simulink model "BoostConverter11_5V_616976422"  (R2017a)
settings: Solver=VariableStepAuto  StartTime=0.0  StopTime=0.1  MaxStep=1e-4  RelTol=1e-3
undefined symbols (not defined in the file): Imag, Real
libraries: powerlib x12
settings Model: Creator=Weliwaththa's - ROG  LastModifiedBy=Weliwaththa's - ROG

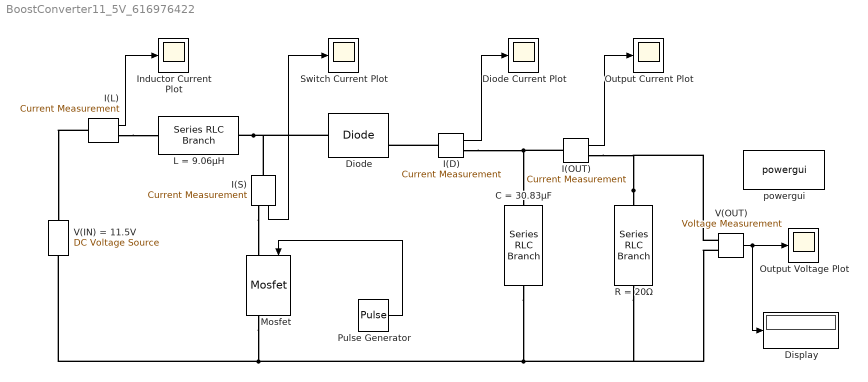
== system BoostConverter11_5V_616976422 ==
  C = 30.83µF : powerlib/Elements/Series RLC Branch  LConnTagsString=__new0  RConnTagsString=__new0  BranchType=C  Resistance=1  Inductance=1e-3  SetiL0=off  InitialCurrent=0  Capacitance=30.83e-6  Setx0=off  InitialVoltage=0  Measurements=None
  Diode : powerlib/Power Electronics/Diode  Ron=0.001  Lon=0  Vf=0.8  IC=0  UseSnubber=0  Rs=500  Cs=250e-9  Measurements=on
  Diode Current Plot : Scope
  Display : Display
  I(D) : powerlib/Measurements/Current Measurement  PhasorSimulation=off  OutputType=Complex  PSBequivalent=0
  I(L) : powerlib/Measurements/Current Measurement  PhasorSimulation=off  OutputType=Real-Imag  PSBequivalent=0
  I(OUT) : powerlib/Measurements/Current Measurement  PhasorSimulation=off  OutputType=Complex  PSBequivalent=0
  I(S) : powerlib/Measurements/Current Measurement  PhasorSimulation=off  OutputType=Complex  PSBequivalent=0
  Inductor Current Plot : Scope
  L = 9.06µH : powerlib/Elements/Series RLC Branch  LConnTagsString=__new0  RConnTagsString=__new0  BranchType=L  Resistance=1  Inductance=9.06e-6  SetiL0=off  InitialCurrent=0  Capacitance=1e-6  Setx0=off  InitialVoltage=0  Measurements=None
  Mosfet : powerlib/Power Electronics/Mosfet  Ron=0  Lon=0  Rd=0  Vfd=0  IC=0  Rs=1e5  Cs=inf  Measurements=on
  Output Current Plot : Scope
  Output Voltage Plot : Scope
  Pulse Generator : DiscretePulseGenerator  PulseType=Time based  Period=1e-5  PulseWidth=61.67
  R = 20Ω : powerlib/Elements/Series RLC Branch  LConnTagsString=__new0  RConnTagsString=__new0  BranchType=R  Resistance=20  Inductance=1e-3  SetiL0=off  InitialCurrent=0  Capacitance=1e-6  Setx0=off  InitialVoltage=0  Measurements=None
  Switch Current Plot : Scope
  V(IN) = 11.5V : powerlib/Electrical Sources/DC Voltage Source  Amplitude=11.5  Measurements=Voltage
  V(OUT) : powerlib/Measurements/Voltage Measurement  PhasorSimulation=off  OutputType=Complex  PSBequivalent=0
  powergui : powerlib/powergui  Priority=1  SimulationMode=Continuous  SampleTime=50e-6  frequency=60  Iterations=50  frequencyindice=0  Pbase=100e6  ErrMax=1e-4  UnitsV=kV  UnitsW=MW  buscounter=0  FunctionMessages=off  echomessages=off  EnableUseOfTLC=off  CurrentSourceSwitches=off  DisableSnubberDevices=off  DisableRonSwitches=off  DisableVfSwitches=off  DisplayEquations=off  SolverType=Tustin/Backward Euler (TBE)  Interpol=off  ExternalGateDelay=off  methode=off  Ts=100  x0status=blocks  SPID=on  SwTol=0  HookPort=off  RestoreLinks=warning  ResistiveCurrentMeasurement=off  Frange=[0:2:500]  Ylog=off  Xlog=on  ShowGrid=off  save=off  variable=ZData  structure=0  ZoomFFT=off  StartTime=0.0  cycles=1  DisplayStyle=1  fundamental=60  FreqAxis=off  MaxFrequency=1000  frequencyindicesteady=1  RmsSteady=1  display=off
  wires:
  I(S)/1 -> Switch Current Plot/1
  I(OUT)/1 -> Output Current Plot/1
  I(L)/1 -> Inductor Current Plot/1
  V(OUT)/1 -> Output Voltage Plot/1, Display/1
  I(D)/1 -> Diode Current Plot/1
  Pulse Generator/1 -> Mosfet/1
  connections:
  I(D)/RConn1 -- I(OUT)/LConn1 -- C = 30.83µF/LConn1
  V(OUT)/LConn2 -- R = 20Ω/RConn1 -- C = 30.83µF/RConn1 -- Mosfet/RConn1 -- V(IN) = 11.5V/LConn1
  I(L)/LConn1 -- V(IN) = 11.5V/RConn1
  L = 9.06µH/RConn1 -- I(S)/LConn1 -- Diode/LConn1
  R = 20Ω/LConn1 -- V(OUT)/LConn1 -- I(OUT)/RConn1
  I(D)/LConn1 -- Diode/RConn1
  I(L)/RConn1 -- L = 9.06µH/LConn1
  I(S)/RConn1 -- Mosfet/LConn1
